simulink model "fxpdemo_integrate"  (Simulink 5.0)
settings: Solver=ode5  SolverMode=SingleTasking  StartTime=0.0  StopTime=4  FixedStep=SampleTime/5  RelTol=1e-3  AbsTol=1e-6
PreLoadFcn:
  | preload_integrate
InitFcn:
  | ;
StartFcn:
  | ;
StopFcn:
  | ;
values from neighbouring files (symbols this model uses):
  SampleTime = 0.05    [preload_integrate.m]    (also in preload_lead_lag.m; preload_state_space.m = 0.01)
libraries: fixpt_lib_4 x8, fixpt_lib_3p1 x1
PreSaveFcn:
  | ;
settings Model: CovMetricSettings=d  MinMaxOverflowLogging=MinMaxAndOverflow  Creator=andyb  LastModifiedBy=andyb  ExtModeTrigMode=oneshot  ExtModeArmWhenConnect=off  ExtModeAutoUpdateStatusClock=off  TimeSaveName=timetest  OutputSaveName=youttest  LimitDataPoints=off  IntegerOverflowMsg=none  ParameterDowncastMsg=warning  ParameterOverflowMsg=warning  ParameterPrecisionLossMsg=none  BooleanDataType=off  RTWOptions="-aRollThreshold=5 -aShowEliminatedStatements=1 -aRTWVerbose=1 -aLocalBlockOutputs=1 -aInlineInvariantSignals=1 -aLogVarNameModifier=\"rt_\""

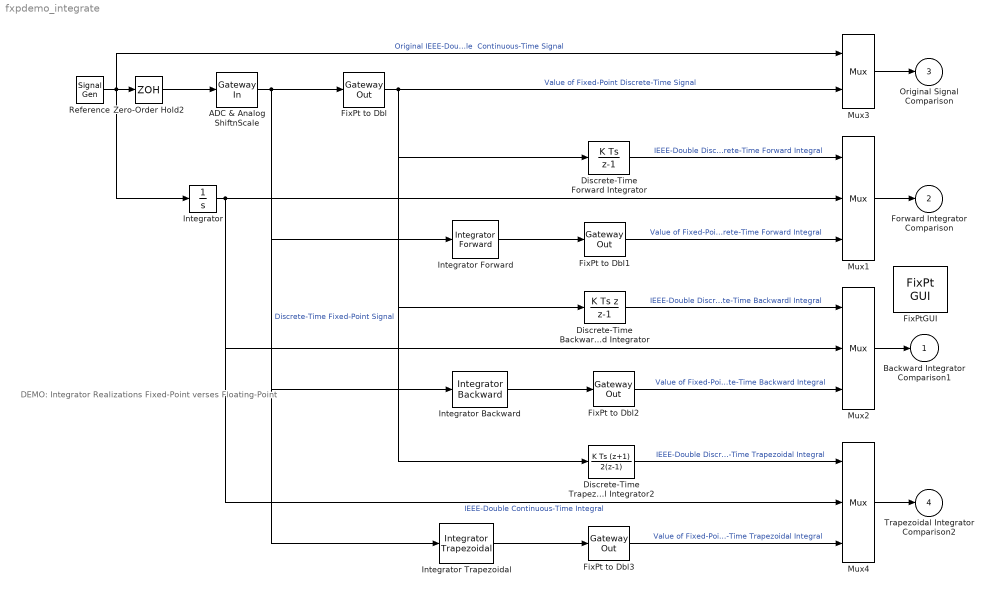
== system fxpdemo_integrate ==
  note: DEMO:
      |
      | Integrator
      | Realizations
      |
      | Fixed-Point
      | verses
      | Floating-Point
  ADC & Analog ShiftnScale : fixpt_lib_4/Data Type/Gateway In  InRealWorld=Real World Value  OutputDataTypeScalingMode=Specify via dialog  OutDataType=sfix(16)  OutScaling=2^-9  RndMeth=Nearest  DoSatur=on
      settings: LockScale=on
  Discrete-Time Backward Integrator : DiscreteIntegrator  IntegratorMethod=Backward Euler  SampleTime=SampleTime
  Discrete-Time Forward Integrator : DiscreteIntegrator  SampleTime=SampleTime
  Discrete-Time Trapezoidal Integrator2 : DiscreteIntegrator  IntegratorMethod=Trapezoidal  SampleTime=SampleTime
  FixPt to Dbl{,1..3} (4 alike) : fixpt_lib_4/Data Type/Gateway Out  OutRealWorld=Real World Value  OutBuiltInType=double  DoSatur=off
  FixPtGUI : fixpt_lib_3p1/FixPt GUI
  Integrator : Integrator
  Integrator Backward : fixpt_lib_4/Calculus/Integrator Backward  gainval=1.0  ICPrevOutput=0.0  OutDataType=sfix(16)  OutScaling=2^-10  DoSatur=off
  Integrator Forward : fixpt_lib_4/Calculus/Integrator Forward  gainval=1.0  ICPrevOutput=0.0  OutDataType=sfix(16)  OutScaling=2^-10  DoSatur=off
  Integrator Trapezoidal : fixpt_lib_4/Calculus/Integrator Trapezoidal  gainval=1.0  ICPrevOutput=0.0  ICPrevScaledInput=0.0  OutDataType=sfix(16)  OutScaling=2^-10  DoSatur=off
  Mux1 : Mux  Inputs=3
  Mux2 : Mux  Inputs=3
  Mux3 : Mux  Inputs=2
  Mux4 : Mux  Inputs=3
  Reference : SignalGenerator  Amplitude=-1  Frequency=0.1*2.5
  Zero-Order Hold2 : ZeroOrderHold  SampleTime=SampleTime
  Backward Integrator Comparison1 : Outport
  Forward Integrator Comparison : Outport  Port=2
  Original Signal Comparison : Outport  Port=3
  Trapezoidal Integrator Comparison2 : Outport  Port=4
  wires:
  Zero-Order Hold2/1 -> ADC & Analog ShiftnScale/1
  ADC & Analog ShiftnScale/1 -> FixPt to Dbl/1, Integrator Forward/1, Integrator Backward/1, Integrator Trapezoidal/1  "Discrete-Time Fixed-Point Signal"
  FixPt to Dbl/1 -> Mux3/2, Discrete-Time Forward Integrator/1, Discrete-Time Backward Integrator/1, Discrete-Time Trapezoidal Integrator2/1  "Value of Fixed-Point Discrete-Time Signal"
  Mux3/1 -> Original Signal Comparison/1
  Reference/1 -> Mux3/1, Integrator/1, Zero-Order Hold2/1  "Original IEEE-Double  Continuous-Time Signal"
  FixPt to Dbl1/1 -> Mux1/3  "Value of Fixed-Point Discrete-Time Forward Integral"
  Mux1/1 -> Forward Integrator Comparison/1
  Discrete-Time Forward Integrator/1 -> Mux1/1  "IEEE-Double Discrete-Time Forward Integral"
  Integrator Forward/1 -> FixPt to Dbl1/1
  Integrator/1 -> Mux1/2, Mux2/2, Mux4/2  "IEEE-Double Continuous-Time Integral"
  FixPt to Dbl2/1 -> Mux2/3  "Value of Fixed-Point Discrete-Time Backward Integral"
  Mux2/1 -> Backward Integrator Comparison1/1
  Discrete-Time Backward Integrator/1 -> Mux2/1  "IEEE-Double Discrete-Time Backwardl Integral"
  Integrator Backward/1 -> FixPt to Dbl2/1
  FixPt to Dbl3/1 -> Mux4/3  "Value of Fixed-Point Discrete-Time Trapezoidal Integral"
  Mux4/1 -> Trapezoidal Integrator Comparison2/1
  Discrete-Time Trapezoidal Integrator2/1 -> Mux4/1  "IEEE-Double Discrete-Time Trapezoidal Integral"
  Integrator Trapezoidal/1 -> FixPt to Dbl3/1
